simulink model "commadaptivemimo"  (R2018b)
settings: Solver=FixedStepDiscrete  StartTime=0.0  StopTime=inf  RelTol=1e-3  EnableMultiTasking=on
PreLoadFcn:
  | adaptivemimo.FrameLen=120;
  | adaptivemimo.SNR=10;
  | adaptivemimo.TargetFER=2e-1;
  | adaptivemimo.MaxNumErrs=500;
  | adaptivemimo.MaxNumFrames=5e6;
undefined symbols (not defined in the file): doppler
libraries: commdigbbndpm3 x2, dspindex x2, commvarsize x1, commrandsrc3 x1, commsink2 x1, commblksprivate x1, commchan3 x1
CloseFcn:
  | blk='commadaptivemimo/Visualization';
  | gfig = findobj('type', 'figure', 'tag', blk);
  | close(gfig);
  | clear blk gfig;
Description:
  | Adaptive MIMO System with OSTBC
  | 
  | This model shows an adaptive orthogonal space-time block code (OSTBC) transceiver system over a multiple-input multiple-output (MIMO) channel.
settings Model: FPTRunName=Active  Creator=The MathWorks, Inc.  LastModifiedBy=nhj94
settings DataIOCC: LimitDataPoints=on  SaveFormat=Array
settings OptimizationCC: BlockReduction=off  ConditionallyExecuteInputs=off  ExpressionDepthLimit=2147483647  RollThreshold=2  LifeSpan=inf  SimCompilerOptimization=on
settings DebuggingCC: UnderspecifiedInitializationDetection=Classic  MergeDetectMultiDrivingBlocksExec=none  FcnCallInpInsideContextMsg=warning  AllowSymbolicDim=off  StateNameClashWarn=warning  SFUnexpectedBacktrackingDiag=warning  SFNoUnconditionalDefaultTransitionDiag=warning  SFExecutionAtInitializationDiag=none
settings HardwareCC: ProdBitPerPointer=32  ProdBitPerSizeT=32  ProdBitPerPtrDiffT=32  ProdLargestAtomicFloat=None  ProdIntDivRoundTo=Undefined  ProdEndianess=Unspecified  ProdWordSize=32  ProdHWDeviceType=32-bit Generic
settings ModelReferenceCC: PropagateSignalLabelsOutOfModel=off
settings SFSimCC: SimUseLocalCustomCode=off  SimParseCustomCode=off
settings RTWCC: RTWUseLocalCustomCode=off  RTWCompilerOptimization=on
settings CodeAppCC: StateflowObjectComments=on
settings GRTTargetCC: TargetLangStandard=C89/C90 (ANSI)  GeneratePreprocessorConditionals=Disable all  CombineOutputUpdateFcns=off  GRTInterface=on
settings ConfigComp: CovMetricSettings=dw  CovHtmlReporting=on  CovSaveCumulativeToWorkspaceVar=on  CovSaveSingleToWorkspaceVar=on  CovExternalEMLEnable=off  CovSFcnEnable=off

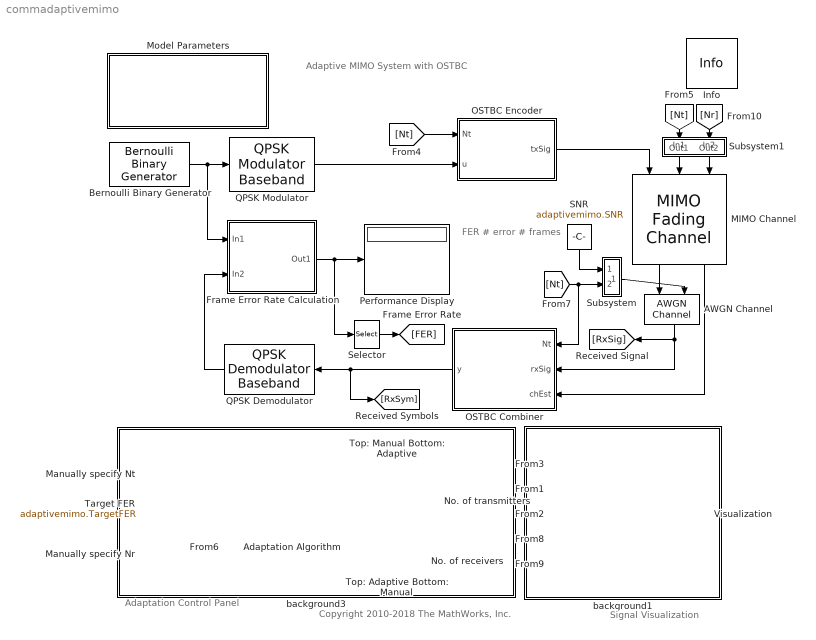
== system commadaptivemimo ==
  note: Adaptive MIMO System with OSTBC
  note: FER
      |
      | # error
      |
      | # frames
  note: Adaptation Control Panel
  note: Signal Visualization
  note: Copyright 2010-2018 The MathWorks, Inc.
  AWGN Channel : commvarsize/AWGN Channel  NoiseMethod=Variance  EbNo=10  EsNo=10  SNR=10  BitsPerSymbol=1  SignalPower=1  SamplesPerSymbol=1  VarianceSource=Input port  Variance=1  RandomStream=mt19937ar with seed  Seed=67  SimulateUsing=Interpreted execution
      settings: SourceProductName=Communications Toolbox  SourceProductBaseCode=CM
  Adaptation Algorithm : Subsystem
  Bernoulli Binary Generator : commrandsrc3/Bernoulli Binary Generator  ProbabilityOfZero=0.5  SeedSource=Parameter  Seed=61  SampleTime=1e-6  SamplesPerFrame=adaptivemimo.FrameLen  OutputDataType=boolean  SimulateUsing=Interpreted execution
      settings: SourceProductName=Communications Toolbox
  Frame Error Rate Calculation : Subsystem
      mask Display: disp('Frame Error Rate\nCalculation');
  Info : commblksprivate/Info  SystemSampleTime=-1
      settings: SourceProductName=Communications Toolbox  SourceProductBaseCode=CM
  MIMO Channel : commchan3/MIMO Fading Channel  InheritSampleRate=off  SampleRate=2e6/3  PathDelays=0  AveragePathGains=0  NormalizePathGains=on  FadingDistribution=Rayleigh  KFactor=3  DirectPathDopplerShift=0  DirectPathInitialPhase=0  MaximumDopplerShift=100  DopplerSpectrum=doppler( 'Jakes' )  SpatialCorrelationSpecification=None  SpatialCorrelationMatrix=[1 0 0 0; 0 1 0 0; 0 0 1 0; 0 0 0 1]  NumTransmitAntennas=4  NumReceiveAntennas=4  TransmitCorrelationMatrix=[1 0; 0 1]  ReceiveCorrelationMatrix=[1 0; 0 1]  AntennaSelection=Tx and Rx  NormalizeChannelOutputs=on  SimulateUsing=Interpreted execution  FadingTechnique=Filtered Gaussian noise  NumSinusoids=48  InitialTimeSource=Property  InitialTime=0  ChannelInterpolationMethod=Polyphase  RandomStream=mt19937ar with seed  Seed=73  PathGainsOutputPort=on  Visualization=Off  AntennaPairsToDisplay=[ 1, 1 ]  PathsForDopplerDisplay=1  SamplesToDisplay=25%
      settings: SourceProductName=Communications Toolbox  SourceProductBaseCode=CM
  Manually specify Nr : Constant  OutDataTypeStr=double
  Manually specify Nt : Constant  Value=2  OutDataTypeStr=double
  Model Parameters : Subsystem  mask(Model Parameters){FrameLen=120, SNR=10, TargetFER=2e-1, MaxNumErrs=500, MaxNumFrames=5e6}
      mask prompts: FrameLen "Frame length:"; SNR "Signal to noise ratio (dB):"; TargetFER "Target frame error rate:"; MaxNumErrs "Maximum number of errors:"; MaxNumFrames "Maximum number of frames:"
      mask help: Load model parameters in MATLAB workspace.
      mask init:
      | mystr=['adaptivemimo.SNR=',num2str(SNR),';'];
      | mystr=[mystr,['adaptivemimo.FrameLen=',num2str(FrameLen),';']];
      | mystr=[mystr,['adaptivemimo.TargetFER=',num2str(TargetFER),';']];
      | mystr=[mystr,['adaptivemimo.MaxNumErrs=',num2str(MaxNumErrs),';']];
      | mystr=[mystr,['adaptivemimo.MaxNumFrames=',num2str(MaxNumFrames),';']];
      | evalin('base',mystr);
      mask Help: helpview(commdhelp);
      mask Display:
      | disp(['Frame length                  ' num2str(FrameLen,'%7.0f')  ...
      | sprintf('\n') 'SNR (dB)                           ' num2str(SNR,'%7.0f') ...
      | sprintf('\n') 'Target FER             ' num2str(TargetFER,'%1.1d')  ...
      | sprintf('\n') 'Max. error count             ' num2str(MaxNumErrs,'%7.0f')  ...
      | sprintf('\n') 'Max. frame count     ' num2str(MaxNumFrames,'%7.0g')]);
  OSTBC Combiner : MATLAB Function  TreatAsAtomicUnit=on
  OSTBC Encoder : MATLAB Function  TreatAsAtomicUnit=on
  Performance Display : Display
  QPSK Demodulator : commdigbbndpm3/QPSK Demodulator Baseband  OutType=Bit  DecType=Hard decision  VarSource=Dialog  Variance=1  Dec=Gray  Ph=0  outDtype1=boolean  outDtype2=Inherit via internal rule  derotateFactorWordLen=16  derotateFactorDataTypeStr=Inherit: Same word length as input  derotateFactorLastDataTypeStr=Inherit: Same word length as input
      settings: SourceProductName=Communications Toolbox
  QPSK Modulator : commdigbbndpm3/QPSK Modulator Baseband  InType=Bit  Enc=Gray  Ph=0  outDtype=double  outWordLen=16  outUDDataType=sfix(16)  outFracLenMode=Best precision  outFracLen=15  outDataTypeStr=double  outLastDataTypeStr=double
      settings: SourceProductName=Communications Toolbox
  SNR : Constant  Value=adaptivemimo.SNR  OutDataTypeStr=double
  Selector : Selector  InputPortWidth=3  IndexOptions=Index vector (dialog)  Indices=1  OutputSizes=1
  Subsystem : Subsystem
  Subsystem1 : Subsystem
  Target FER : Constant  Value=adaptivemimo.TargetFER  OutDataTypeStr=double
  Top: Adaptive Bottom: Manual : ManualSwitch
  Top: Manual Bottom: Adaptive : ManualSwitch  CurrentSetting=0
  Visualization : Subsystem
      settings: OpenFcn=|
      | blk=gcb;
      | gfig = findobj('type', 'figure', 'tag', blk);
      | if isempty(gfig)
      |         gfig = openfig('commadaptivemimo');
      |         set(gfig, 'tag', blk);
      | else
      |     close(gfig);
      | end
      mask Display: disp('Signal\nVisualization\n\nDouble-click to\nopen/close')
  background1 : Subsystem
      mask Display: disp('')
  background3 : Subsystem
      mask Display: disp('')
  wires:
  QPSK Modulator/1 -> OSTBC Encoder/2(u)
  [Nt] -> OSTBC Encoder/1(Nt)
  Target FER/1 -> Adaptation Algorithm/1(Target_FER)
  Adaptation Algorithm/1(Nt) -> Top: Manual Bottom: Adaptive/2
  Top: Manual Bottom: Adaptive/1 -> [Nt]
  [FER] -> Adaptation Algorithm/2(Actual_FER)
  Adaptation Algorithm/2(Nr) -> Top: Adaptive Bottom: Manual/1
  Top: Adaptive Bottom: Manual/1 -> [Nr]
  Manually specify Nt/1 -> Top: Manual Bottom: Adaptive/1
  Manually specify Nr/1 -> Top: Adaptive Bottom: Manual/2
  Selector/1 -> [FER]
  OSTBC Combiner/1(y) -> [RxSym], QPSK Demodulator/1
  [FER] -> Visualization/1(In6)
  [Nt] -> Visualization/2(In7)
  [Nr] -> Visualization/3(In8)
  [RxSig] -> Visualization/4(In9)
  [RxSym] -> Visualization/5(In10)
  Frame Error Rate Calculation/1(Out1) -> Performance Display/1, Selector/1
  QPSK Demodulator/1 -> Frame Error Rate Calculation/2(In2)
  [Nt] -> Subsystem1/1(In1)
  [Nr] -> Subsystem1/2(In2)
  OSTBC Encoder/1(txSig) -> MIMO Channel/1
  Subsystem1/1(Out1) -> MIMO Channel/2
  Subsystem1/2(Out2) -> MIMO Channel/3
  MIMO Channel/2 -> OSTBC Combiner/3(chEst)
  MIMO Channel/1 -> AWGN Channel/1
  AWGN Channel/1 -> OSTBC Combiner/2(rxSig), [RxSig]
  Subsystem/1(Noise Variance) -> AWGN Channel/2
  [Nt] -> OSTBC Combiner/1(Nt), Subsystem/2(In2)
  SNR/1 -> Subsystem/1(In1)
  Bernoulli Binary Generator/1 -> QPSK Modulator/1, Frame Error Rate Calculation/1(In1)

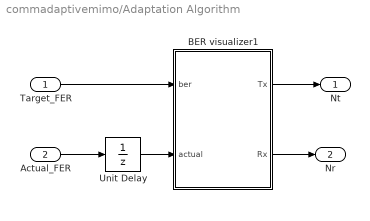
== system commadaptivemimo/Adaptation Algorithm ==
  Target_FER : Inport
  Actual_FER : Inport  Port=2
  BER visualizer1 : MATLAB Function  TreatAsAtomicUnit=on
  Unit Delay : UnitDelay  InitialCondition=1  SampleTime=-1
  Nt : Outport
  Nr : Outport  Port=2
  wires:
  Unit Delay/1 -> BER visualizer1/2(actual)
  Actual_FER/1 -> Unit Delay/1
  Target_FER/1 -> BER visualizer1/1(ber)
  BER visualizer1/1(Tx) -> Nt/1
  BER visualizer1/2(Rx) -> Nr/1

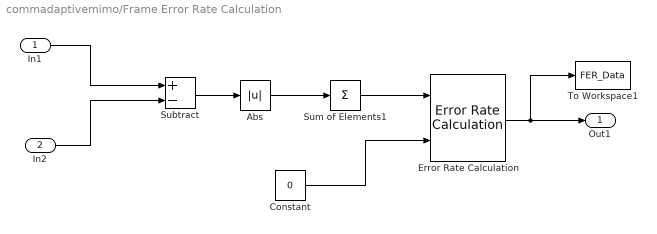
== system commadaptivemimo/Frame Error Rate Calculation ==
  In1 : Inport
  In2 : Inport  Port=2
  Abs : Abs
  Constant : Constant  Value=0  OutDataTypeStr=uint16
  Error Rate Calculation : commsink2/Error Rate Calculation  N=0  st_delay=0  cp_mode=Entire frame  subframe=[]  PMode=Port  WsName=FERdata  RsMode2=off  stop=on  numErr=adaptivemimo.MaxNumErrs  maxBits=adaptivemimo.MaxNumFrames
      settings: SourceProductName=Communications Toolbox
  Subtract : Sum  Inputs=+-  AccumDataTypeStr=int8  OutDataTypeStr=int8
  Sum of Elements1 : Sum  Inputs=+  AccumDataTypeStr=uint16  OutDataTypeStr=uint16  SaturateOnIntegerOverflow=on
  To Workspace1 : ToWorkspace  VariableName=FER_Data  SampleTime=-1
      settings: MaxDataPoints=1
  Out1 : Outport
  wires:
  Error Rate Calculation/1 -> Out1/1, To Workspace1/1
  Constant/1 -> Error Rate Calculation/2
  Sum of Elements1/1 -> Error Rate Calculation/1
  Abs/1 -> Sum of Elements1/1
  Subtract/1 -> Abs/1
  In2/1 -> Subtract/2
  In1/1 -> Subtract/1

== system commadaptivemimo/Model Parameters ==

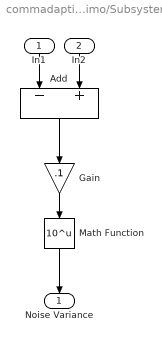
== system commadaptivemimo/Subsystem ==
  In1 : Inport
  In2 : Inport  Port=2
  Add : Sum  Inputs=-+
  Gain : Gain  Gain=.1
  Math Function : Math  Operator=10^u  SaturateOnIntegerOverflow=on
  Noise Variance : Outport
  wires:
  In1/1 -> Add/1
  In2/1 -> Add/2
  Math Function/1 -> Noise Variance/1
  Gain/1 -> Math Function/1
  Add/1 -> Gain/1

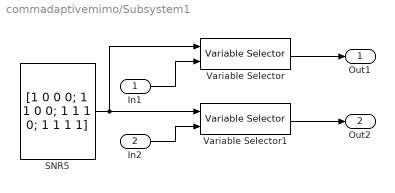
== system commadaptivemimo/Subsystem1 ==
  In1 : Inport
  In2 : Inport  Port=2
  SNR5 : Constant  Value=[1 0 0 0; 1 1 0 0; 1 1 1 0; 1 1 1 1]  VectorParams1D=off  OutDataTypeStr=double
  Variable Selector : dspindex/Variable Selector  NumInputs=1  rowsOrCols=Rows  IdxMode=Variable  Elements=[1 3]  ZerOneIdxMode=One-based  errmode=Clip Index  FillMode=on  FillValues=0
  Variable Selector1 : dspindex/Variable Selector  NumInputs=1  rowsOrCols=Rows  IdxMode=Variable  Elements=[1 3]  ZerOneIdxMode=One-based  errmode=Clip Index  FillMode=on  FillValues=0
  Out1 : Outport
  Out2 : Outport  Port=2
  wires:
  Variable Selector/1 -> Out1/1
  SNR5/1 -> Variable Selector/1, Variable Selector1/1
  In2/1 -> Variable Selector1/2
  Variable Selector1/1 -> Out2/1
  In1/1 -> Variable Selector/2

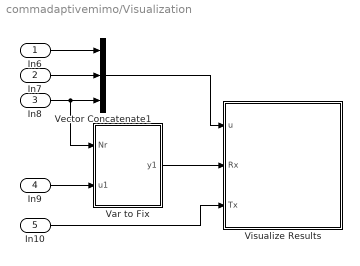
== system commadaptivemimo/Visualization ==
  In6 : Inport
  In7 : Inport  Port=2
  In8 : Inport  Port=3
  In9 : Inport  Port=4
  In10 : Inport  Port=5
  Var to Fix : MATLAB Function  TreatAsAtomicUnit=on
  Vector Concatenate1 : Concatenate  NumInputs=3
  Visualize Results : MATLAB Function  TreatAsAtomicUnit=on
  wires:
  Vector Concatenate1/1 -> Visualize Results/1(u)
  In6/1 -> Vector Concatenate1/1
  In9/1 -> Var to Fix/2(u1)
  In7/1 -> Vector Concatenate1/2
  In8/1 -> Vector Concatenate1/3, Var to Fix/1(Nr)
  In10/1 -> Visualize Results/3(Tx)
  Var to Fix/1(y1) -> Visualize Results/2(Rx)

== system commadaptivemimo/background1 ==

== system commadaptivemimo/background3 ==

== matlab function commadaptivemimo/OSTBC Combiner ==
  data: Nt input; y output size=[adaptivemimo.FrameLen/2 1]; rxSig input size=[2*adaptivemimo.FrameLen/3  4]; chEst input size=[2*adaptivemimo.FrameLen/3 1 4 4]; adaptivemimo parameter size=[1,1]
function y = ostbc_combiner(Nt, rxSig, chEst, adaptivemimo)
%#codegen

persistent h2Tx1Rx h2Tx2Rx h2Tx3Rx h2Tx4Rx h3Tx1Rx h3Tx2Rx h3Tx3Rx h3Tx4Rx h4Tx1Rx h4Tx2Rx h4Tx3Rx h4Tx4Rx
if isempty(h2Tx1Rx)
    h2Tx1Rx = comm.OSTBCCombiner('NumTransmitAntennas', 2, 'NumReceiveAntennas',  1);
    h2Tx2Rx = comm.OSTBCCombiner('NumTransmitAntennas', 2, 'NumReceiveAntennas',  2);
    h2Tx3Rx = comm.OSTBCCombiner('NumTransmitAntennas', 2, 'NumReceiveAntennas',  3);
    h2Tx4Rx = comm.OSTBCCombiner('NumTransmitAntennas', 2, 'NumReceiveAntennas',  4);
    h3Tx1Rx = comm.OSTBCCombiner('NumTransmitAntennas', 3, 'NumReceiveAntennas',  1);
    h3Tx2Rx = comm.OSTBCCombiner('NumTransmitAntennas', 3, 'NumReceiveAntennas',  2);
    h3Tx3Rx = comm.OSTBCCombiner('NumTransmitAntennas', 3, 'NumReceiveAntennas',  3);
    h3Tx4Rx = comm.OSTBCCombiner('NumTransmitAntennas', 3, 'NumReceiveAntennas',  4);
    h4Tx1Rx = comm.OSTBCCombiner('NumTransmitAntennas', 4, 'NumReceiveAntennas',  1);
    h4Tx2Rx = comm.OSTBCCombiner('NumTransmitAntennas', 4, 'NumReceiveAntennas',  2);
    h4Tx3Rx = comm.OSTBCCombiner('NumTransmitAntennas', 4, 'NumReceiveAntennas',  3);
    h4Tx4Rx = comm.OSTBCCombiner('NumTransmitAntennas', 4, 'NumReceiveAntennas',  4);
end

Nr = size(rxSig, 2);
channelEst = squeeze(chEst(:,1,:,:));

switch Nt
    case 1 % MRC
        chEst1Tx = squeeze(channelEst(:,1,1:Nr));
        yTemp = sum(rxSig(:,1:Nr) .* conj(chEst1Tx), 2) / norm(chEst1Tx, 'fro')^2;
    case 2
        switch Nr
        case 1
            yTemp = step(h2Tx1Rx, rxSig(:,1),   channelEst(:,1:2,1));
        case 2
            yTemp = step(h2Tx2Rx, rxSig(:,1:2), channelEst(:,1:2,1:2));
        case 3
            yTemp = step(h2Tx3Rx, rxSig(:,1:3), channelEst(:,1:2,1:3));
        otherwise % Nr == 4
            yTemp = step(h2Tx4Rx, rxSig(:,1:4), channelEst(:,1:2,1:4));
        end
    case 3
        switch Nr
        case 1
            yTemp = step(h3Tx1Rx, rxSig(:,1),   channelEst(:,1:3,1));
        case 2
            yTemp = step(h3Tx2Rx, rxSig(:,1:2), channelEst(:,1:3,1:2));
        case 3
            yTemp = step(h3Tx3Rx, rxSig(:,1:3), channelEst(:,1:3,1:3));
        otherwise % Nr == 4
            yTemp = step(h3Tx4Rx, rxSig(:,1:4), channelEst(:,1:3,1:4));
        end
    otherwise % Nt = 4
        switch Nr
        case 1
            yTemp = step(h4Tx1Rx, rxSig(:,1),   channelEst(:,1:4,1));
        case 2
            yTemp = step(h4Tx2Rx, rxSig(:,1:2), channelEst(:,1:4,1:2));
        case 3
            yTemp = step(h4Tx3Rx, rxSig(:,1:3), channelEst(:,1:4,1:3));
        otherwise % Nr == 4
            yTemp = step(h4Tx4Rx, rxSig(:,1:4), channelEst(:,1:4,1:4));
        end
end

y = yTemp(1:adaptivemimo.FrameLen/2, 1);

== matlab function commadaptivemimo/OSTBC Encoder ==
  data: Nt input size=[1,1]; u input size=[adaptivemimo.FrameLen/2 1]; txSig output size=[2*adaptivemimo.FrameLen/3  4]
function txSig = ostbc_encoder(Nt, u)
%#codegen

persistent h2Tx h3Tx h4Tx
if isempty(h2Tx)
    h2Tx = comm.OSTBCEncoder('NumTransmitAntennas', 2);
    h3Tx = comm.OSTBCEncoder('NumTransmitAntennas', 3);
    h4Tx = comm.OSTBCEncoder('NumTransmitAntennas', 4);    
end

switch Nt
    case 2
        txSig = step(h2Tx, u);
    case 3
        txSig = step(h3Tx, u);
    case 4
        txSig = step(h4Tx, u);
    otherwise % numTx = 1
        txSig = u;
end
end

== matlab function commadaptivemimo/Visualization/Var to Fix ==
  data: Nr input; u1 input size=[2*adaptivemimo.FrameLen/3  4]; y1 output size=[2*adaptivemimo.FrameLen/3  4]; adaptivemimo parameter
function y1 =var2fix(Nr, u1,adaptivemimo)
%#codegen
FrameLen=adaptivemimo.FrameLen;
y1=complex(nan(2*FrameLen/3,4));
for n=1:Nr
    y1(1:size(u1,1),n)=u1(:,n);
end

== matlab function commadaptivemimo/Visualization/Visualize Results ==
  data: u input size=3; Rx input; Tx input
function VisualizeMe(u,Rx,Tx)
%#codegen
 N=300;  
persistent fc ber
if isempty(fc)
    fc=1;
    ber=nan(N,1);
end
%
coder.extrinsic('findobj','axes','semilogy','bar',      'set','plot');
%
if ~strcmp(coder.target, 'rtw') 
    gfig = findobj('type', 'figure', 'tag', 'commadaptivemimo/Visualization');
    if isempty(gfig)
        fc=1;
    else
        ax1 = findobj('type', 'axes', 'tag','MyBer');
        ax2 = findobj('type', 'axes', 'tag','MyRate');
        
        axTx1 = findobj('type', 'axes', 'tag','RxSym');
        
        axRx1 = findobj('type', 'axes', 'tag','MyRx1');
        axRx2 = findobj('type', 'axes', 'tag','MyRx2');
        axRx3 = findobj('type', 'axes', 'tag','MyRx3');
        axRx4 = findobj('type', 'axes', 'tag','MyRx4');
        
        ber(N)=u(1);
        Rate=[u(2) u(3)];
        %% Update plots using handles
        if fc
            % 1st plot FER as a function of frames
            semilogy(ax1,1:N,ber,'dr');
            % 2nd plot Number of Tx and Rx
            bar(ax2,Rate,'b');
            % Received symbols
            plot(axTx1,Tx,'.b');
            % Rx constellations
            plot(axRx1,Rx(:,1),'.b');
            plot(axRx2,Rx(:,2),'.b');
            plot(axRx3,Rx(:,3),'.b');
            plot(axRx4,Rx(:,4),'.b');
        else
            % 1st plot FER as a function of frames
            c = get(ax1, 'child');
            set(c, 'ydata', ber);
            % 2nd plot Number of Tx and Rx
            c = get(ax2, 'child');
            set(c, 'xdata', [ 1 2]);
            set(c, 'ydata', Rate);
            % Received symbols
            c = get(axTx1, 'child');
            set(c, 'xdata', real(Tx));
            set(c, 'ydata', imag(Tx));
            % Rx constelattions
            c = get(axRx1, 'child');
            set(c, 'xdata', real(Rx(:,1)));
            set(c, 'ydata', imag(Rx(:,1)));
            c = get(axRx2, 'child');
            set(c, 'xdata', real(Rx(:,2)));
            set(c, 'ydata', imag(Rx(:,2)));
            c = get(axRx3, 'child');
            set(c, 'xdata', real(Rx(:,3)));
            set(c, 'ydata', imag(Rx(:,3)));
            c = get(axRx4, 'child');
            set(c, 'xdata', real(Rx(:,4)));
            set(c, 'ydata', imag(Rx(:,4)));
        end
        %% Update the states
        ber(1:N-1)=ber(2:N);
        fc=0;
    end
end

== matlab function commadaptivemimo/Adaptation Algorithm/BER visualizer1 ==
  data: Tx output size=1; Rx output size=1; ber input; actual input
function [Tx,Rx]=Adaptation(ber,actual)
%#codegen
mu=0.2;
persistent v
if isempty(v)
    v=[1 1];
end
Tx=fix(v(1));
Rx=fix(v(2));
err=actual-ber;
v=v+mu*([0.9 1.1].*sign(err));
v(v<1)=1;
v(v>4)=4;
